simulink model "simTPDA1"  (R2013a)
settings: Solver=ode3  StartTime=0.0  StopTime=20  FixedStep=tSampling  RelTol=1e-3
values from neighbouring files (symbols this model uses):
  Tb = eye(4)    [T_basic.m]    (also in main_via_point.m)
undefined symbols (not defined in the file or in its folder): bDevice, bWall, DBPf, DBPv, DiscIntNeverNeededParam, filterON, kc, Kp, Kv, kWall, mc, mDevice, nWall, POPCM_off, POPCS_off, posCompensation, randTime, sigbuilder_block, T1, Tf, tSampling, v0Device, xDevice, xWall
libraries: simulink x1
settings Model: Creator=thaole910  LastModifiedBy=thaole910

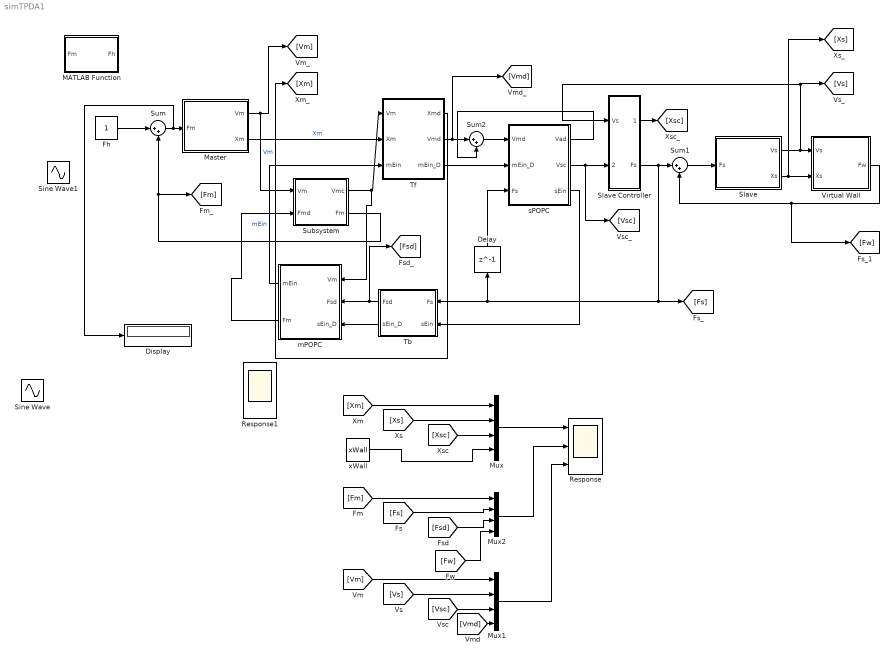
== system simTPDA1 ==
  Delay : Delay  DelayLength=1  InitialCondition=0  SampleTime=tSampling
  Display : Display
  Fh : Constant
  MATLAB Function : MATLAB Function  TreatAsAtomicUnit=on
  Master : Subsystem
  Mux : Mux
  Mux1 : Mux
  Mux2 : Mux
  Response : Scope  NumInputPorts=3
      settings: ShowLegends=on  TimeRange=4.291187739463602  YMin=-3~-500~-150  YMax=1~150~175  Decimation=10  SampleInput=on
  Response1 : Scope  NumInputPorts=3
      settings: ShowLegends=on  TimeRange=0.3838709677419353  YMin=-45~-0.5~-1  YMax=10~1.5~1  Decimation=10  SampleInput=on
  Sine Wave : Sin  Amplitude=1.5  Frequency=10  SampleTime=0
  Sine Wave1 : Sin  Bias=1  Frequency=5  SampleTime=0
  Slave : Subsystem
  Slave Controller : Subsystem
  Subsystem : Subsystem
  Sum : Sum  Inputs=|++
  Sum1 : Sum  Inputs=|++
  Sum2 : Sum  Inputs=|++
  Tb : Subsystem
  Tf : Subsystem
  Virtual Wall : Subsystem
  mPOPC : Subsystem
  sPOPC : Subsystem
  xWall : Constant  Value=xWall
  wires:
  Tb/1(Fsd) -> [Fsd], mPOPC/2(Fsd)
  sPOPC/2(Vsc) -> [Vsc], Slave Controller/2(Vsc)
  sPOPC/3(sEin) -> Tb/2(sEin)
  Slave/1(Vs) -> [Vs], Slave Controller/1(Vs), Virtual Wall/1(Vs)
  Master/1(Vm) -> Subsystem/1(Vm), [Vm]  "Vm"
  mPOPC/1(mEin) -> Tf/3(mEin)  "mEin"
  Slave/2(Xs) -> [Xs], Virtual Wall/2(Xs)
  Sum1/1 -> Slave/1(Fs)
  Slave Controller/1(Xsc) -> [Xsc]
  [Xm] -> Mux/1
  [Xs] -> Mux/2
  [Xsc] -> Mux/3
  xWall/1 -> Mux/4
  [Fm] -> Mux2/1
  [Fs] -> Mux2/2
  [Fsd] -> Mux2/3
  [Vm] -> Mux1/1
  [Vs] -> Mux1/2
  [Vsc] -> Mux1/3
  Mux/1 -> Response/1
  Mux2/1 -> Response/2
  Mux1/1 -> Response/3
  [Vmd] -> Mux1/4
  Tf/3(mEin_D) -> sPOPC/2(mEin_D)
  Tb/2(sEin_D) -> mPOPC/3(sEin_D)
  [Fw] -> Mux2/4
  Tf/1(Xmd) -> [Xm]
  Slave Controller/2(Fs) -> Delay/1, Tb/1(Fs), [Fs], Sum1/1
  Sum/1 -> Display/1, Master/1(Fm)
  Sum2/1 -> sPOPC/1(Vmd)
  Tf/2(Vmd) -> [Vmd], Sum2/1
  sPOPC/1(Vad) -> Sum2/2
  Virtual Wall/1(Fw) -> Sum1/2, [Fw]
  Delay/1 -> sPOPC/3(Fs)
  Master/2(Xm) -> Tf/2(Xm)  "Xm"
  Subsystem/1(Vmc) -> mPOPC/1(Vm), Tf/1(Vm)
  mPOPC/2(Fm) -> Subsystem/2(Fmd)
  Subsystem/2(Fm) -> [Fm], Sum/2
  Fh/1 -> Sum/1

== system simTPDA1/Master ==
  Fm : Inport
  Integrator : Integrator  InitialCondition=v0Device  UpperSaturationLimit=10  LowerSaturationLimit=-10
  Integrator1 : Integrator  InitialCondition=xDevice  UpperSaturationLimit=10  LowerSaturationLimit=-10
  Sum : Sum  Inputs=|+-
  "b " : Gain  Gain=bDevice
  b 1 : Gain  Gain=1/mDevice
  Vm : Outport
  Xm : Outport  Port=2
  wires:
  b 1/1 -> Integrator/1
  Fm/1 -> Sum/1
  "b "/1 -> Sum/2
  Sum/1 -> b 1/1
  Integrator/1 -> "b "/1, Vm/1, Integrator1/1
  Integrator1/1 -> Xm/1

== system simTPDA1/Slave ==
  Fs : Inport
  Integrator : Integrator  InitialCondition=v0Device  UpperSaturationLimit=10  LowerSaturationLimit=-10
  Integrator1 : Integrator  InitialCondition=xDevice  UpperSaturationLimit=10  LowerSaturationLimit=-10
  Sum : Sum  Inputs=|+-
  "b " : Gain  Gain=bDevice
  b 1 : Gain  Gain=1/mDevice
  Vs : Outport
  Xs : Outport  Port=2
  wires:
  b 1/1 -> Integrator/1
  Fs/1 -> Sum/1
  "b "/1 -> Sum/2
  Sum/1 -> b 1/1
  Integrator/1 -> "b "/1, Vs/1, Integrator1/1
  Integrator1/1 -> Xs/1

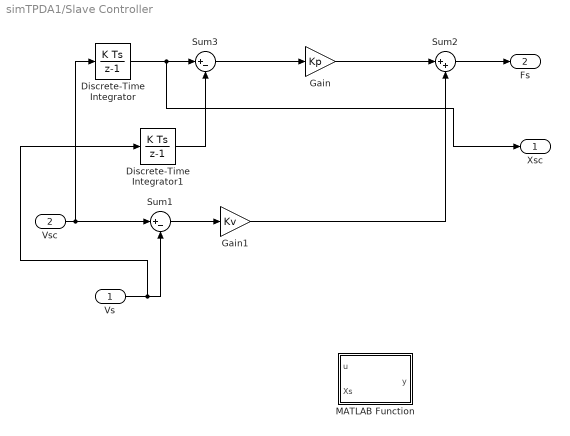
== system simTPDA1/Slave Controller ==
  Vs : Inport
  Vsc : Inport  Port=2
  Discrete-Time Integrator : DiscreteIntegrator  SampleTime=tSampling  ICPrevOutput=DiscIntNeverNeededParam  ICPrevScaledInput=DiscIntNeverNeededParam
  Discrete-Time Integrator1 : DiscreteIntegrator  SampleTime=tSampling  ICPrevOutput=DiscIntNeverNeededParam  ICPrevScaledInput=DiscIntNeverNeededParam
  Gain : Gain  Gain=Kp
  Gain1 : Gain  Gain=Kv
  MATLAB Function : MATLAB Function  TreatAsAtomicUnit=on
  Sum1 : Sum  Inputs=|+-
  Sum2 : Sum  Inputs=|++
  Sum3 : Sum  Inputs=|+-
  Xsc : Outport
  Fs : Outport  Port=2
  wires:
  Sum1/1 -> Gain1/1
  Gain/1 -> Sum2/1
  Vs/1 -> Discrete-Time Integrator1/1, Sum1/2
  Sum2/1 -> Fs/1
  Sum3/1 -> Gain/1
  Vsc/1 -> Sum1/1, Discrete-Time Integrator/1
  Discrete-Time Integrator/1 -> Xsc/1, Sum3/1
  Discrete-Time Integrator1/1 -> Sum3/2
  Gain1/1 -> Sum2/2

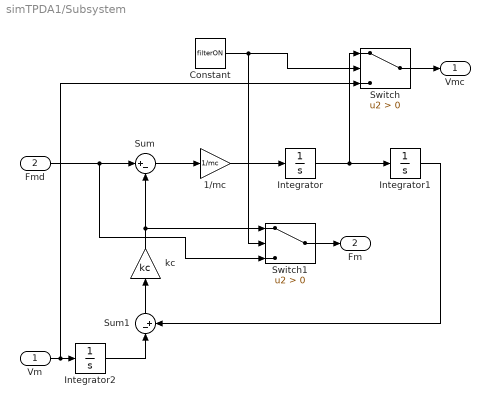
== system simTPDA1/Subsystem ==
  Vm : Inport
  Fmd : Inport  Port=2
  1/mc : Gain  Gain=1/mc
  Constant : Constant  Value=filterON
  Integrator : Integrator
  Integrator1 : Integrator
  Integrator2 : Integrator
  Sum : Sum  Inputs=|+-
  Sum1 : Sum  Inputs=|-+
  Switch : Switch  Criteria=u2 > Threshold
  Switch1 : Switch  Criteria=u2 > Threshold
  kc : Gain  Gain=kc
  Vmc : Outport
  Fm : Outport  Port=2
  wires:
  Fmd/1 -> Switch1/3, Sum/1
  Sum/1 -> 1/mc/1
  Integrator/1 -> Switch/1, Integrator1/1
  Sum1/1 -> kc/1
  kc/1 -> Sum/2, Switch1/1
  Integrator1/1 -> Sum1/2
  1/mc/1 -> Integrator/1
  Switch/1 -> Vmc/1
  Vm/1 -> Switch/3, Integrator2/1
  Integrator2/1 -> Sum1/1
  Switch1/1 -> Fm/1
  Constant/1 -> Switch1/2, Switch/2

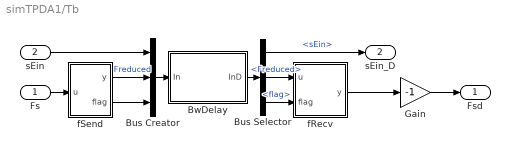
== system simTPDA1/Tb ==
  Fs : Inport
  sEin : Inport  Port=2
  Bus Creator : BusCreator  Inputs=3
  Bus Selector : BusSelector  OutputSignals=sEin,Freduced,flag
  BwDelay : Subsystem
  Gain : Gain  Gain=-1
  fRecv : Subsystem
  fSend : Subsystem
  Fsd : Outport
  sEin_D : Outport  Port=2
  wires:
  fSend/1(y) -> Bus Creator/2  "Freduced"
  Bus Creator/1 -> BwDelay/1(In)
  Bus Selector/2 -> fRecv/1(u)  "<Freduced>"
  Fs/1 -> fSend/1(u)
  fRecv/1(y) -> Gain/1
  Bus Selector/3 -> fRecv/2(flag)  "<flag>"
  fSend/2(flag) -> Bus Creator/3
  BwDelay/1(InD) -> Bus Selector/1
  sEin/1 -> Bus Creator/1
  Bus Selector/1 -> sEin_D/1  "<sEin>"
  Gain/1 -> Fsd/1

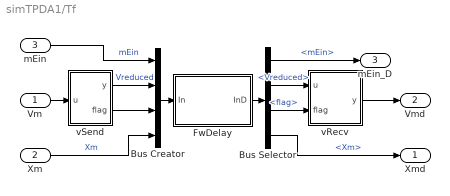
== system simTPDA1/Tf ==
  Vm : Inport
  Xm : Inport  Port=2
  mEin : Inport  Port=3
  Bus Creator : BusCreator
  Bus Selector : BusSelector  OutputSignals=mEin,Vreduced,flag,Xm
  FwDelay : Subsystem
  vRecv : Subsystem
  vSend : Subsystem
  Xmd : Outport
  Vmd : Outport  Port=2
  mEin_D : Outport  Port=3
  wires:
  vSend/1(y) -> Bus Creator/2  "Vreduced"
  Bus Creator/1 -> FwDelay/1(In)
  mEin/1 -> Bus Creator/1  "mEin"
  Vm/1 -> vSend/1(u)
  vRecv/1(y) -> Vmd/1
  Bus Selector/3 -> vRecv/2(flag)  "<flag>"
  vSend/2(flag) -> Bus Creator/3
  FwDelay/1(InD) -> Bus Selector/1
  Bus Selector/1 -> mEin_D/1  "<mEin>"
  Bus Selector/2 -> vRecv/1(u)  "<Vreduced>"
  Xm/1 -> Bus Creator/4  "Xm"
  Bus Selector/4 -> Xmd/1  "<Xm>"

== system simTPDA1/Virtual Wall ==
  Vs : Inport
  Xs : Inport  Port=2
  Demux : Demux
  Force Response : MATLAB Function  TreatAsAtomicUnit=on
  VirtualWall : Constant  Value=[xWall kWall bWall nWall]  VectorParams1D=off
  Fw : Outport
  wires:
  Force Response/1(fWall) -> Fw/1
  Vs/1 -> Force Response/2(Vs)
  Demux/1 -> Force Response/3(xWall)
  Demux/2 -> Force Response/4(kWall)
  Demux/3 -> Force Response/5(bWall)
  Demux/4 -> Force Response/6(nWall)
  VirtualWall/1 -> Demux/1
  Xs/1 -> Force Response/1(Xs)

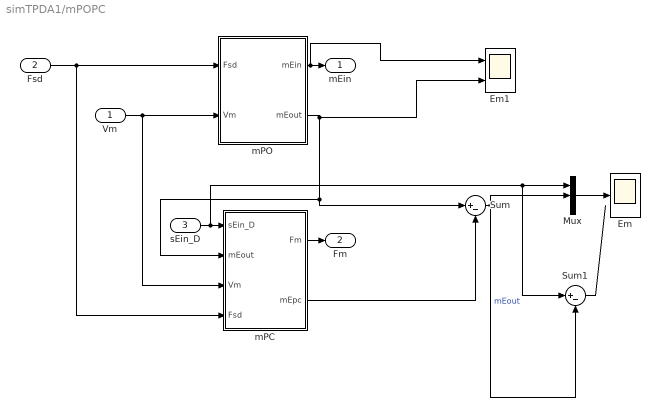
== system simTPDA1/mPOPC ==
  Vm : Inport
  Fsd : Inport  Port=2
  sEin_D : Inport  Port=3
  Em : Scope
      settings: ShowLegends=on  TimeRange=0.8967741935483869  YMin=8.25e+06  YMax=8.725e+06  SaveName=F
  Em1 : Scope  NumInputPorts=2
      settings: ShowLegends=on  TimeRange=0.8967741935483869  YMin=8.25e+06~-5  YMax=8.725e+06~5  SaveName=F2
  Mux : Mux  Inputs=3
  Sum : Sum  Inputs=|+-
  Sum1 : Sum  Inputs=|+-
  mPC : Subsystem
  mPO : Subsystem
  mEin : Outport
  Fm : Outport  Port=2
  wires:
  Fsd/1 -> mPC/4(Fsd), mPO/1(Fsd)
  mPC/1(Fm) -> Fm/1
  Vm/1 -> mPO/2(Vm), mPC/3(Vm)
  Mux/1 -> Em/1
  sEin_D/1 -> Sum1/1, Mux/1, mPC/1(sEin_D)
  mPO/2(mEout) -> Em1/2, Sum/1, mPC/2(mEout)
  mPC/2("mEpc ") -> Sum/2
  Sum/1 -> Sum1/2, Mux/2  "mEout"
  Sum1/1 -> ?
  mPO/1(mEin) -> Em1/1, mEin/1

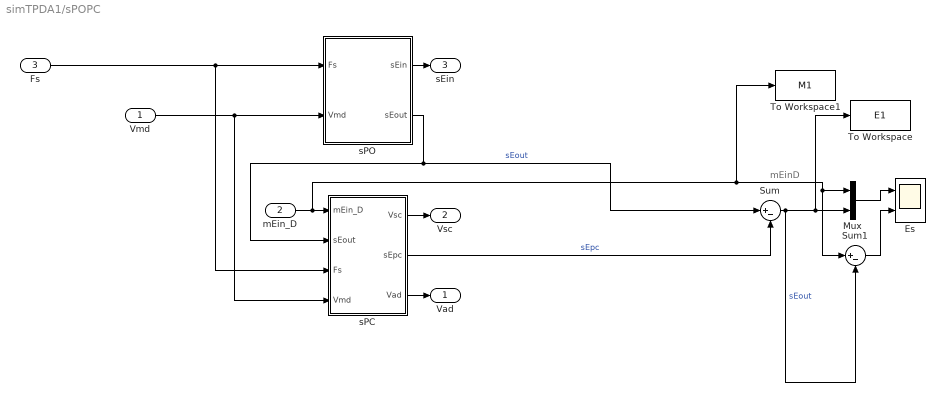
== system simTPDA1/sPOPC ==
  note: mEinD
  Vmd : Inport
  mEin_D : Inport  Port=2
  Fs : Inport  Port=3
  Es : Scope  NumInputPorts=2
      settings: ShowLegends=on  TimeRange=20  YMin=0~-500  YMax=19000~7000  SaveName=F1
  Mux : Mux  Inputs=3
  Sum : Sum  Inputs=|+-
  Sum1 : Sum  Inputs=|+-
  To Workspace : ToWorkspace  VariableName=E1  SampleTime=-1  SaveFormat=Timeseries
  To Workspace1 : ToWorkspace  VariableName=M1  SampleTime=-1  SaveFormat=Timeseries
  sPC : Subsystem
  sPO : Subsystem
  Vad : Outport
  Vsc : Outport  Port=2
  sEin : Outport  Port=3
  wires:
  Vmd/1 -> sPC/4(Vmd), sPO/2(Vmd)
  sPO/1(sEin) -> sEin/1
  sPO/2(sEout) -> Sum/1, sPC/2(sEout)  "sEout"
  sPC/1(Vsc) -> Vsc/1
  Fs/1 -> sPC/3(Fs), sPO/1(Fs)
  mEin_D/1 -> To Workspace1/1, Sum1/1, Mux/1, sPC/1(mEin_D)
  Mux/1 -> Es/1
  sPC/2(sEpc) -> Sum/2  "sEpc"
  Sum/1 -> Sum1/2, To Workspace/1, Mux/3  "sEout"
  Sum1/1 -> Es/2
  sPC/3(Vad) -> Vad/1

== system simTPDA1/Tb/BwDelay ==
  In : Inport
  randDelay : Subsystem
  InD : Outport
  wires:
  In/1 -> randDelay/1(in)
  randDelay/1(inD) -> InD/1

== system simTPDA1/Tb/fRecv ==
  u : Inport
  flag : Inport  Port=2
  Forward delay4 : Delay  DelayLength=1  InitialCondition=0  InputProcessing=Inherited  SampleTime=tSampling
  MATLAB Function : MATLAB Function  TreatAsAtomicUnit=on
  y : Outport
  wires:
  MATLAB Function/1(ik) -> y/1, Forward delay4/1
  Forward delay4/1 -> MATLAB Function/2(ik_1)
  u/1 -> MATLAB Function/1(ik_red)
  flag/1 -> MATLAB Function/3(flag)

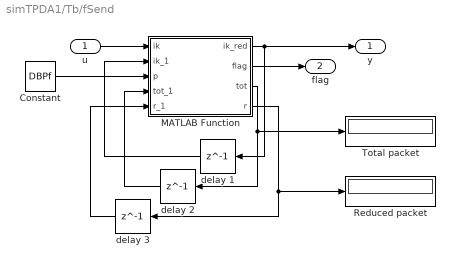
== system simTPDA1/Tb/fSend ==
  u : Inport
  Constant : Constant  Value=DBPf
  MATLAB Function : MATLAB Function  TreatAsAtomicUnit=on
  Reduced packet : Display
  Total packet : Display
  delay 1 : Delay  DelayLength=1  InitialCondition=0  InputProcessing=Inherited  SampleTime=tSampling
  delay 2 : Delay  DelayLength=1  InitialCondition=0  InputProcessing=Inherited  SampleTime=tSampling
  delay 3 : Delay  DelayLength=1  InitialCondition=0  InputProcessing=Inherited  SampleTime=tSampling
  y : Outport
  flag : Outport  Port=2
  wires:
  MATLAB Function/1(ik_red) -> delay 1/1, y/1
  delay 1/1 -> MATLAB Function/2(ik_1)
  Constant/1 -> MATLAB Function/3(p)
  u/1 -> MATLAB Function/1(ik)
  MATLAB Function/2(flag) -> flag/1
  MATLAB Function/3(tot) -> delay 2/1, Total packet/1
  delay 2/1 -> MATLAB Function/4(tot_1)
  MATLAB Function/4(r) -> Reduced packet/1, delay 3/1
  delay 3/1 -> MATLAB Function/5(r_1)

== system simTPDA1/Tf/FwDelay ==
  In : Inport
  randDelay : Subsystem
  InD : Outport
  wires:
  In/1 -> randDelay/1(in)
  randDelay/1(inD) -> InD/1

== system simTPDA1/Tf/vRecv ==
  u : Inport
  flag : Inport  Port=2
  Forward delay4 : Delay  DelayLength=1  InitialCondition=0  InputProcessing=Inherited  SampleTime=tSampling
  MATLAB Function : MATLAB Function  TreatAsAtomicUnit=on
  y : Outport
  wires:
  MATLAB Function/1(ik) -> y/1, Forward delay4/1
  Forward delay4/1 -> MATLAB Function/2(ik_1)
  u/1 -> MATLAB Function/1(ik_red)
  flag/1 -> MATLAB Function/3(flag)

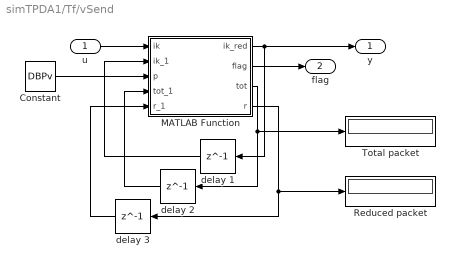
== system simTPDA1/Tf/vSend ==
  u : Inport
  Constant : Constant  Value=DBPv
  MATLAB Function : MATLAB Function  TreatAsAtomicUnit=on
  Reduced packet : Display
  Total packet : Display
  delay 1 : Delay  DelayLength=1  InitialCondition=0  InputProcessing=Inherited  SampleTime=tSampling
  delay 2 : Delay  DelayLength=1  InitialCondition=0  InputProcessing=Inherited  SampleTime=tSampling
  delay 3 : Delay  DelayLength=1  InitialCondition=0  InputProcessing=Inherited  SampleTime=tSampling
  y : Outport
  flag : Outport  Port=2
  wires:
  MATLAB Function/1(ik_red) -> delay 1/1, y/1
  delay 1/1 -> MATLAB Function/2(ik_1)
  Constant/1 -> MATLAB Function/3(p)
  u/1 -> MATLAB Function/1(ik)
  MATLAB Function/2(flag) -> flag/1
  MATLAB Function/3(tot) -> delay 2/1, Total packet/1
  delay 2/1 -> MATLAB Function/4(tot_1)
  MATLAB Function/4(r) -> Reduced packet/1, delay 3/1
  delay 3/1 -> MATLAB Function/5(r_1)

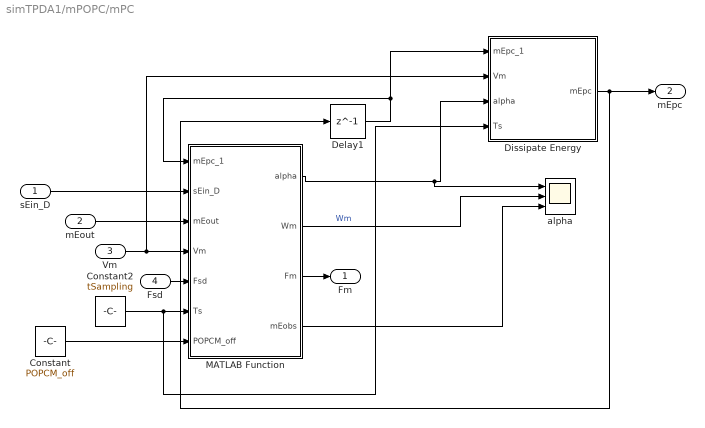
== system simTPDA1/mPOPC/mPC ==
  sEin_D : Inport
  mEout : Inport  Port=2
  Vm : Inport  Port=3
  Fsd : Inport  Port=4
  Constant : Constant  Value=POPCM_off
  Constant2 : Constant  Value=tSampling
  Delay1 : Delay  DelayLength=1  InitialCondition=0  InputProcessing=Inherited  SampleTime=tSampling
  Dissipate Energy : MATLAB Function  TreatAsAtomicUnit=on
  MATLAB Function : MATLAB Function  TreatAsAtomicUnit=on
  alpha : Scope  NumInputPorts=3
      settings: TimeRange=10  YMin=-1~0~-5  YMax=8~3.5~5  SaveName=ScopeData3
  Fm : Outport
  "mEpc " : Outport  Port=2
  wires:
  sEin_D/1 -> MATLAB Function/2(sEin_D)
  Vm/1 -> MATLAB Function/4(Vm), Dissipate Energy/2(Vm)
  Dissipate Energy/1(mEpc) -> Delay1/1, "mEpc "/1
  mEout/1 -> MATLAB Function/3(mEout)
  MATLAB Function/3(Fm) -> Fm/1
  Fsd/1 -> MATLAB Function/5(Fsd)
  Constant2/1 -> Dissipate Energy/4(Ts), MATLAB Function/6(Ts)
  Delay1/1 -> Dissipate Energy/1(mEpc_1), MATLAB Function/1(mEpc_1)
  Constant/1 -> MATLAB Function/7(POPCM_off)
  MATLAB Function/1(alpha) -> alpha/1, Dissipate Energy/3(alpha)
  MATLAB Function/2(Wm) -> alpha/2  "Wm"
  MATLAB Function/4(mEobs) -> alpha/3

== system simTPDA1/mPOPC/mPO ==
  Fsd : Inport
  Vm : Inport  Port=2
  Constant : Constant  Value=tSampling
  Delay : Delay  DelayLength=1  InitialCondition=0  InputProcessing=Inherited  SampleTime=tSampling
  Delay1 : Delay  DelayLength=1  InitialCondition=0  InputProcessing=Inherited  SampleTime=tSampling
  m : MATLAB Function  TreatAsAtomicUnit=on
  mEin : Outport
  mEout : Outport  Port=2
  wires:
  Delay1/1 -> m/4(mEout_1)
  Constant/1 -> m/5(Ts)
  m/2(mEout) -> Delay1/1, mEout/1
  Delay/1 -> m/3(mEin_1)
  m/1(mEin) -> mEin/1, Delay/1
  Fsd/1 -> m/1(Fsd)
  Vm/1 -> m/2(Vm)

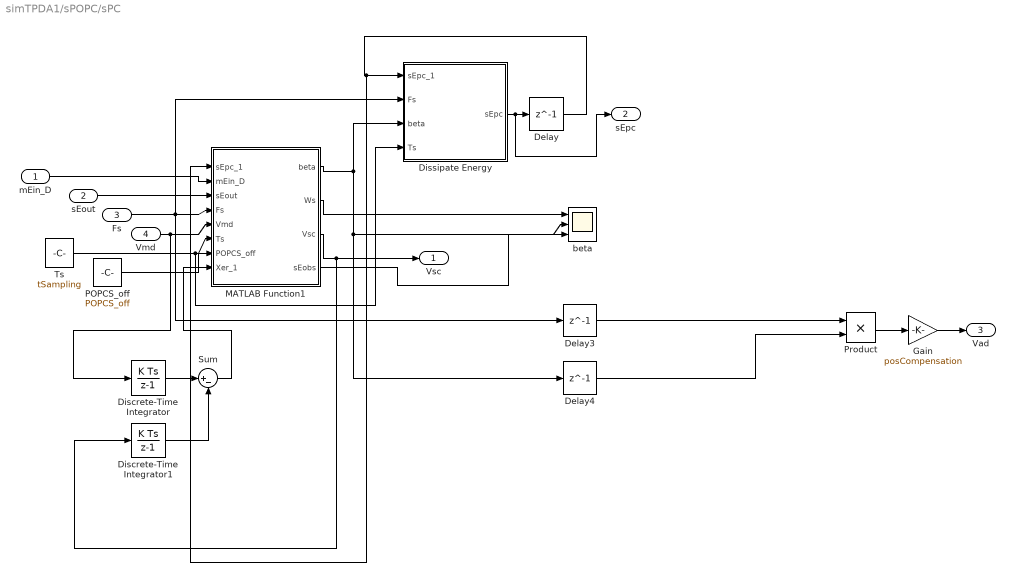
== system simTPDA1/sPOPC/sPC ==
  mEin_D : Inport
  sEout : Inport  Port=2
  Fs : Inport  Port=3
  Vmd : Inport  Port=4
  Delay : Delay  DelayLength=1  InitialCondition=0  InputProcessing=Inherited  SampleTime=tSampling
  Delay3 : Delay  DelayLength=1  InitialCondition=0  InputProcessing=Inherited  SampleTime=tSampling
  Delay4 : Delay  DelayLength=1  InitialCondition=0  InputProcessing=Inherited  SampleTime=tSampling
  Discrete-Time Integrator : DiscreteIntegrator  SampleTime=tSampling  ICPrevOutput=DiscIntNeverNeededParam  ICPrevScaledInput=DiscIntNeverNeededParam
  Discrete-Time Integrator1 : DiscreteIntegrator  SampleTime=tSampling  ICPrevOutput=DiscIntNeverNeededParam  ICPrevScaledInput=DiscIntNeverNeededParam
  Dissipate Energy : MATLAB Function  TreatAsAtomicUnit=on
  Gain : Gain  Gain=posCompensation
  MATLAB Function1 : MATLAB Function  TreatAsAtomicUnit=on
  POPCS_off : Constant  Value=POPCS_off
  Product : Product
  Sum : Sum  Inputs=|+-
  Ts : Constant  Value=tSampling
  beta : Scope  NumInputPorts=3
      settings: TimeRange=0.01147242455775244  YMin=-100~0~-5  YMax=300~15000~5  SaveName=ScopeData4
  Vsc : Outport
  sEpc : Outport  Port=2
  Vad : Outport  Port=3
  wires:
  MATLAB Function1/3(Vsc) -> Discrete-Time Integrator1/1, Vsc/1
  Fs/1 -> Delay3/1, MATLAB Function1/4(Fs), Dissipate Energy/2(Fs)
  mEin_D/1 -> MATLAB Function1/2(mEin_D)
  Ts/1 -> Dissipate Energy/4(Ts), MATLAB Function1/6(Ts)
  Vmd/1 -> Discrete-Time Integrator/1, MATLAB Function1/5(Vmd)
  sEout/1 -> MATLAB Function1/3(sEout)
  Dissipate Energy/1(sEpc) -> sEpc/1, Delay/1
  POPCS_off/1 -> MATLAB Function1/7(POPCS_off)
  Delay/1 -> MATLAB Function1/1(sEpc_1), Dissipate Energy/1(sEpc_1)
  MATLAB Function1/2(Ws) -> beta/1
  Discrete-Time Integrator/1 -> Sum/1
  Discrete-Time Integrator1/1 -> Sum/2
  Sum/1 -> MATLAB Function1/8(Xer_1)
  Gain/1 -> Vad/1
  Product/1 -> Gain/1
  Delay4/1 -> Product/2
  Delay3/1 -> Product/1
  MATLAB Function1/1(beta) -> Delay4/1, beta/2, Dissipate Energy/3(beta)
  MATLAB Function1/4(sEobs) -> beta/3

== system simTPDA1/sPOPC/sPO ==
  Fs : Inport
  Vmd : Inport  Port=2
  Constant1 : Constant  Value=tSampling
  Delay2 : Delay  DelayLength=1  InitialCondition=0  InputProcessing=Inherited  SampleTime=tSampling
  Delay3 : Delay  DelayLength=1  InitialCondition=0  InputProcessing=Inherited  SampleTime=tSampling
  s : MATLAB Function  TreatAsAtomicUnit=on
  sEin : Outport
  sEout : Outport  Port=2
  wires:
  s/2(sEout) -> Delay3/1, sEout/1
  Delay2/1 -> s/3(sEin_1)
  Constant1/1 -> s/5(Ts)
  Delay3/1 -> s/4(sEout_1)
  s/1(sEin) -> sEin/1, Delay2/1
  Fs/1 -> s/1(Fs)
  Vmd/1 -> s/2(Vmd)

== system simTPDA1/Tb/BwDelay/randDelay ==
  in : Inport
  Constant : Constant  Value=Tb
  Constant1 : Constant  Value=randTime
  Delay : Delay  DelayLengthSource=Input port  DelayLength=T1  DelayLengthUpperLimit=Tb  InitialCondition=0  SampleTime=tSampling
      settings: InputPortMap=u0,p1
  Scope : Scope
      settings: YMin=-12.49956  YMax=112.49995  SaveName=ScopeData6
  Sine Wave : Sin  Amplitude=Tb  Bias=Tb+1  SampleTime=tSampling
  Switch : Switch  Criteria=u2 ~= 0
  inD : Outport
  wires:
  in/1 -> Delay/1
  Delay/1 -> inD/1
  Constant/1 -> Switch/3
  Switch/1 -> Delay/2, Scope/1
  Constant1/1 -> Switch/1, Switch/2

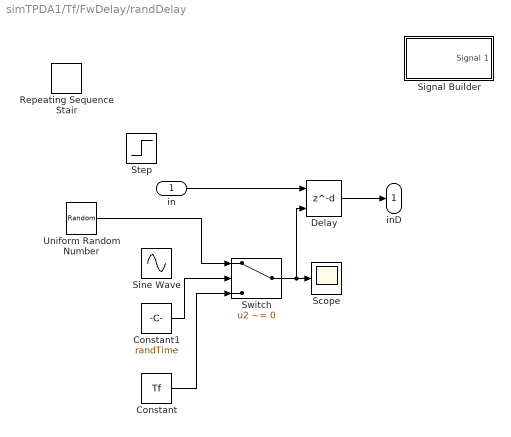
== system simTPDA1/Tf/FwDelay/randDelay ==
  in : Inport
  Constant : Constant  Value=Tf
  Constant1 : Constant  Value=randTime
  Delay : Delay  DelayLengthSource=Input port  DelayLength=T1  DelayLengthUpperLimit=5000  InitialCondition=0  SampleTime=tSampling
      settings: InputPortMap=u0,p1
  Repeating Sequence Stair : simulink/Sources/Repeating Sequence Stair  OutValues=[10 600].'  tsamp=tSampling  OutMin=[]  OutMax=[]  OutDataTypeStr=double  OutputDataTypeScalingMode=double  OutDataType=fixdt(0,8)  ConRadixGroup=Best Precision: Vector-wise  OutScaling=2^-12
  Scope : Scope
      settings: YMin=-93.75  YMax=843.75  SaveName=ScopeData6
  Signal Builder : Subsystem  Tag=STV Subsys  LoadFcn=sigbuilder_block('load');  StartFcn=sigbuilder_block('start');  StopFcn=sigbuilder_block('stop');  ClipboardFcn=sigbuilder_block('clipboard');  mask(Sigbuilder block){}
      mask help: Simulink:masks:SigbuilderBlock_MD
      mask init:
      | if ~strcmp(get_param(bdroot(gcbh),'SimulationStatus'),'stopped') tuvar = sigbuilder_block('maskInit'); end
      settings: CopyFcn=sigbuilder_block('copy');  DeleteFcn=sigbuilder_block('delete');  ModelCloseFcn=sigbuilder_block('modelClose');  PreSaveFcn=sigbuilder_block('preSave');  PauseFcn=sigbuilder_block('pause');  ContinueFcn=sigbuilder_block('continue');  NameChangeFcn=sigbuilder_block('namechange');  OpenFcn=sigbuilder_block('open',[0 28.5 1015.5 483.75 ]);  CloseFcn=sigbuilder_block('close');
      mask Display: plot(0, 0, 100, 100,[2, 2, 32, 32, 2], [68, 8, 8, 68, 68],[32, 2], [38, 38], [32, 19, 2],[53, 60, 44], [32, 17, 17, 2],[16, 16, 31, 31]);txt = getActiveGroup(gcbh);text(2, 100, txt,'verticalAlignment', 'top');
  Sine Wave : Sin  Amplitude=Tf  Bias=Tf+1  Frequency=10000  Phase=pi/2  SampleTime=tSampling
  Step : Step  Time=2  Before=100  After=400  SampleTime=0
  Switch : Switch  Criteria=u2 ~= 0
  Uniform Random Number : UniformRandomNumber  Minimum=1  Maximum=Tf+1  SampleTime=tSampling
  inD : Outport
  wires:
  in/1 -> Delay/1
  Delay/1 -> inD/1
  Constant/1 -> Switch/3
  Constant1/1 -> Switch/2
  Switch/1 -> Delay/2, Scope/1
  Uniform Random Number/1 -> Switch/1

== system simTPDA1/Tf/FwDelay/randDelay/Signal Builder ==
  Demux : Demux  Tag=STV Demux  Outputs=1
  FromWs : FromWorkspace  Tag=STV FromWs  VariableName=tuvar  SampleTime=0
      SigBuilderData=|
      | common.afterFinalStr = 'Extrapolate'
      | common.sampleTime = 0
      | dataSet.timeRange = [0 10]
      | dataSet.name = 'Group 1'
      | sbobj.Groups.Name = 'Group 1'
      | sbobj.Groups.Signals.Name = 'Signal 1'
      | sbobj.Groups.Signals.XData = [0 4 4 6 6 10]
      | sbobj.Groups.Signals.YData = [1 1 51 51 100 100]
  Signal 1 : Outport  Tag=STV Outport
  wires:
  Demux/1 -> Signal 1/1
  FromWs/1 -> Demux/1

== matlab function simTPDA1/sPOPC/sPO/s ==
  data: Fs input; sEin output; Vmd input; sEin_1 input; sEout_1 input; Ts input; sEout output
function[sEin,sEout] = fcn(Fs,Vmd,sEin_1,sEout_1,Ts)
dE = Fs*Vmd*Ts;
    if dE > 0
        sEin = sEin_1;
        sEout = sEout_1 + dE;
    else
        sEin = sEin_1 - dE;
        sEout = sEout_1;
    end
end

== matlab function simTPDA1/mPOPC/mPO/m ==
  data: Fsd input; mEin output; Vm input; mEin_1 input; mEout_1 input; Ts input; mEout output
function[mEin,mEout] = fcn(Fsd,Vm,mEin_1,mEout_1,Ts)
dE = -Fsd*Vm*Ts;
    if dE > 0
        mEin = mEin_1 + dE;
        mEout = mEout_1;
    else
        mEin = mEin_1;
        mEout = mEout_1 - dE;
    end
end

== matlab function simTPDA1/Tb/fRecv/MATLAB Function ==
  data: ik output; ik_red input; ik_1 input; flag input
function ik = fcn(ik_red,ik_1,flag)
if flag == 1
   ik = ik_red;
else
   ik = ik_1;
end

== matlab function simTPDA1/sPOPC/sPC/Dissipate Energy ==
  data: sEpc_1 input; sEpc output; Fs input; beta input; Ts input
function sEpc = fcn(sEpc_1,Fs,beta,Ts)
    sEpc = Fs^2*beta*Ts  + sEpc_1;
end

== matlab function simTPDA1/mPOPC/mPC/Dissipate Energy ==
  data: mEpc_1 input; Vm input; alpha input; Ts input; mEpc output
function mEpc = fcn(mEpc_1,Vm,alpha,Ts)
    mEpc =  Vm^2*alpha*Ts + mEpc_1;
end

== matlab function simTPDA1/mPOPC/mPC/MATLAB Function ==
  data: mEpc_1 input; sEin_D input; alpha output; mEout input; Wm output; Vm input; Fsd input; Ts input; Fm output; POPCM_off input; mEobs output
function [alpha,Wm,Fm,mEobs] = fcn(mEpc_1,sEin_D,mEout,Vm,Fsd,Ts,POPCM_off)
    Wm = sEin_D - mEout + mEpc_1;
    if (Wm < 0) && (abs(Vm) > 1e-2)
        alpha = - Wm/(Ts*Vm^2);
    else
        alpha = 0;
    end
    if (POPCM_off)
        alpha = 0;
    end
    Fm = Fsd - alpha*Vm;
    mEobs = Wm + alpha*Vm^2*Ts;
end

== matlab function simTPDA1/sPOPC/sPC/MATLAB Function1 ==
  data: sEpc_1 input; mEin_D input; beta output; sEout input; Ws output; Fs input; Vmd input; Ts input; Vsc output; POPCS_off input; Xer_1 input; sEobs output
function [beta,Ws,Vsc,sEobs] = fcn(sEpc_1,mEin_D,sEout,Fs,Vmd,Ts,POPCS_off,Xer_1)
    Ws = mEin_D - sEout + sEpc_1;
    if (Ws < 0) && (abs(Fs) > 0)
        beta = -Ws/(Ts*Fs^2);
    elseif (abs(Fs) > 0)
        beta = sign(-Xer_1)*min(abs(Xer_1),abs(Ws/Fs))/(Fs*Ts); 
    else
        beta = 0;
    end
    if (POPCS_off)
        beta = 0;
    end
    Vsc = Vmd - beta*Fs;
    sEobs = Ws + beta*Fs^2*Ts;
end

== matlab function simTPDA1/Tb/fSend/MATLAB Function ==
  data: ik input; ik_red output; ik_1 input; p input; flag output; tot_1 input; r_1 input; tot output; r output
function [ik_red,flag,tot,r]= fcn(ik,ik_1,p,tot_1,r_1)
DB = p*abs(ik);
if abs(ik-ik_1) >= DB
    ik_red = ik;
    flag = 1;
    r = r_1;
else
    ik_red = ik_1;
    r = r_1 + 1;
    flag = 0;
end
tot = tot_1 + 1;

== matlab function simTPDA1/Virtual Wall/Force Response ==
  data: Xs input; fWall output; Vs input; xWall input; kWall input; bWall input; nWall input
function fWall = fcn(Xs,Vs,xWall,kWall,bWall,nWall)
if ((Xs-xWall)'*nWall < 0) 
    fWall = -kWall*((Xs-xWall)'*nWall)*nWall - bWall*((Vs'*nWall)*nWall);
    if fWall'*nWall < 0 
        fWall = 0;
    end
else
    fWall =0;
end

== matlab function simTPDA1/Tf/vSend/MATLAB Function ==
  data: ik input; ik_red output; ik_1 input; p input; flag output; tot_1 input; r_1 input; tot output; r output
function [ik_red,flag,tot,r]= fcn(ik,ik_1,p,tot_1,r_1)
DB = p*abs(ik);
if abs(ik-ik_1) >= DB
    ik_red = ik;
    flag = 1;
    r = r_1;
else
    ik_red = ik_1;
    r = r_1 + 1;
    flag = 0;
end
tot = tot_1 + 1;

== matlab function simTPDA1/Slave Controller/MATLAB Function ==
  data: u input; y output; Xs input
function y = fcn(u,Xs)
if Xs > 0.1
    y = 150*u;
else
    y = 3*u;
end

== matlab function simTPDA1/MATLAB Function ==
  data: Fm input; Fh output
function Fh = fcn(Fm)
if Fm == 0
    Fh = 1;
else
    Fh = -Fm+1;
end

== matlab function simTPDA1/Tf/vRecv/MATLAB Function ==
  data: ik output; ik_red input; ik_1 input; flag input
function ik = fcn(ik_red,ik_1,flag)
if flag == 1
   ik = ik_red;
else
   ik = ik_1;
end
